simulink model "ar04_ss1r_adapt"  (R2020a)
settings: Solver=ode45  StartTime=0.0  StopTime=100  FixedStep=SIMstepSize  RelTol=1e-3  EnableMultiTasking=on
settings Model: Creator=MT  LastModifiedBy=MT
settings DataIOCC: LimitDataPoints=on  SaveFormat=Array  SignalLoggingSaveFormat=ModelDataLogs  SaveOutput=off  SignalLogging=off  DSMLogging=off  SaveTime=off  ReturnWorkspaceOutputs=off
settings OptimizationCC: ExpressionDepthLimit=2147483647  LifeSpan=inf
settings DebuggingCC: UnderspecifiedInitializationDetection=Classic  MergeDetectMultiDrivingBlocksExec=none  SolverPrmCheckMsg=warning  FcnCallInpInsideContextMsg=warning  StateNameClashWarn=warning  SFUnexpectedBacktrackingDiag=warning  SFNoUnconditionalDefaultTransitionDiag=warning  SFExecutionAtInitializationDiag=none  ArithmeticOperatorsInVariantConditions=warning
settings HardwareCC: ProdBitPerPointer=32  ProdBitPerSizeT=32  ProdBitPerPtrDiffT=32  ProdLargestAtomicFloat=None  ProdIntDivRoundTo=Undefined  ProdEndianess=Unspecified  ProdWordSize=32  ProdHWDeviceType=32-bit Generic
settings ModelReferenceCC: PropagateSignalLabelsOutOfModel=off
settings SFSimCC: SimUseLocalCustomCode=off  CustomCodeUndefinedFunction=UseInterfaceOnly
settings RTWCC: RTWUseLocalCustomCode=off
settings CodeAppCC: StateflowObjectComments=on
settings GRTTargetCC: TargetLangStandard=C89/C90 (ANSI)  CombineOutputUpdateFcns=off  GRTInterface=on
settings ConfigComp: CovMetricSettings=dw  CovHtmlReporting=on  CovSaveCumulativeToWorkspaceVar=on  CovSaveSingleToWorkspaceVar=on  CovExternalEMLEnable=off

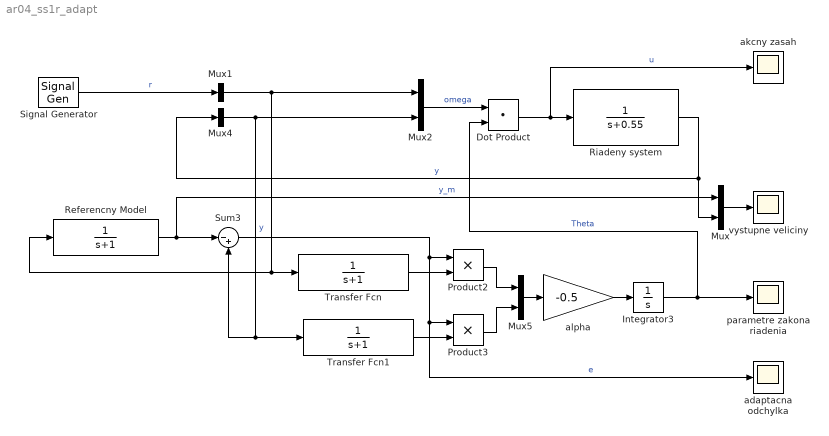
== system ar04_ss1r_adapt ==
  Dot Product : DotProduct  InputSameDT=on  OutDataTypeStr=Inherit: Inherit via internal rule
  Integrator3 : Integrator
  Mux : Mux  Inputs=2
  Mux1 : Mux  Inputs=1
  Mux2 : Mux  Inputs=2
  Mux4 : Mux  Inputs=1
  Mux5 : Mux  Inputs=2
  Product2 : Product  RndMeth=Zero
  Product3 : Product  RndMeth=Zero
  Referencny Model : TransferFcn  Denominator="[1  1]"
  Riadeny system : TransferFcn  Denominator=[1 0.55]
  Signal Generator : SignalGenerator  WaveForm=square  Amplitude=-1  Frequency=1/20
  Sum3 : Sum  Inputs=|-+
  Transfer Fcn : TransferFcn  Denominator=[1 1]
  Transfer Fcn1 : TransferFcn  Denominator=[1 1]
  adaptacna odchylka : Scope
  akcny zasah : Scope
  alpha : Gain  Gain=-0.5
  parametre zakona riadenia : Scope
  vystupne veliciny : Scope
  wires:
  Mux/1 -> vystupne veliciny/1
  Signal Generator/1 -> Mux1/1  "r"
  Referencny Model/1 -> Mux/1, Sum3/1  "y_m"
  Mux1/1 -> Mux2/1, Transfer Fcn/1, Referencny Model/1
  Product2/1 -> Mux5/1
  Product3/1 -> Mux5/2
  Riadeny system/1 -> Mux/2, Mux4/1  "y"
  Mux2/1 -> Dot Product/1  "omega"
  Mux4/1 -> Mux2/2, Transfer Fcn1/1, Sum3/2  "y"
  Transfer Fcn/1 -> Product2/2
  Transfer Fcn1/1 -> Product3/2
  Sum3/1 -> Product2/1, Product3/1, adaptacna odchylka/1  "e"
  Dot Product/1 -> Riadeny system/1, akcny zasah/1  "u"
  Mux5/1 -> alpha/1
  Integrator3/1 -> parametre zakona riadenia/1, Dot Product/2  "Theta"
  alpha/1 -> Integrator3/1
